simulink model "Distribution_v2"  (Simulink 7.9)
settings: Solver=VariableStepDiscrete  StartTime=0.0  StopTime=1000  RelTol=1e-3
libraries: simeventslib x35
(part 5 of 6)

== system Distribution_v2/Customer_15/Commodity_109 ==
  Clock : Clock
  Source : TimeBasedEntityGenerator  Distribution=Exponential  InitialSeed=18340  Mean=Mean  GenerateEntityAtSimulationStart=off
  Timed to Event Signal : TimedToEventSignal
  setAttribute : SetAttribute  AttributeName=Route|Origin|Destination|Start  AttributeFrom=Dialog|Dialog|Dialog|Signal port  AttributeValue="[15  20  11   0]|15|11|1"  AttributeTreatAsVector=0|1|1|1  EvaluatedAttributeValue="{[15  20  11   0];15;11;[]}"
      settings: InputPortMap=u3
  OUT_Commodity : PMIOPort  Port=1  Side=Right
  wires:
  Timed to Event Signal/1 -> setAttribute/1
  Clock/1 -> Timed to Event Signal/1
  connections:
  OUT_Commodity/RConn1 -- setAttribute/RConn1
  Source/RConn1 -- setAttribute/LConn1

== system Distribution_v2/Customer_15/Commodity_110 ==
  Clock : Clock
  Source : TimeBasedEntityGenerator  Distribution=Exponential  InitialSeed=18340  Mean=Mean  GenerateEntityAtSimulationStart=off
  Timed to Event Signal : TimedToEventSignal
  setAttribute : SetAttribute  AttributeName=Route|Origin|Destination|Start  AttributeFrom=Dialog|Dialog|Dialog|Signal port  AttributeValue="[15  20  22  12]|15|12|1"  AttributeTreatAsVector=0|1|1|1  EvaluatedAttributeValue="{[15  20  22  12];15;12;[]}"
      settings: InputPortMap=u3
  OUT_Commodity : PMIOPort  Port=1  Side=Right
  wires:
  Timed to Event Signal/1 -> setAttribute/1
  Clock/1 -> Timed to Event Signal/1
  connections:
  OUT_Commodity/RConn1 -- setAttribute/RConn1
  Source/RConn1 -- setAttribute/LConn1

== system Distribution_v2/Customer_15/Commodity_111 ==
  Clock : Clock
  Source : TimeBasedEntityGenerator  Distribution=Exponential  InitialSeed=18340  Mean=Mean  GenerateEntityAtSimulationStart=off
  Timed to Event Signal : TimedToEventSignal
  setAttribute : SetAttribute  AttributeName=Route|Origin|Destination|Start  AttributeFrom=Dialog|Dialog|Dialog|Signal port  AttributeValue="[15  20  22  13]|15|13|1"  AttributeTreatAsVector=0|1|1|1  EvaluatedAttributeValue="{[15  20  22  13];15;13;[]}"
      settings: InputPortMap=u3
  OUT_Commodity : PMIOPort  Port=1  Side=Right
  wires:
  Timed to Event Signal/1 -> setAttribute/1
  Clock/1 -> Timed to Event Signal/1
  connections:
  OUT_Commodity/RConn1 -- setAttribute/RConn1
  Source/RConn1 -- setAttribute/LConn1

== system Distribution_v2/Customer_2/Commodity_10 ==
  Clock : Clock
  Source : TimeBasedEntityGenerator  Distribution=Exponential  InitialSeed=18340  Mean=Mean  GenerateEntityAtSimulationStart=off
  Timed to Event Signal : TimedToEventSignal
  setAttribute : SetAttribute  AttributeName=Route|Origin|Destination|Start  AttributeFrom=Dialog|Dialog|Dialog|Signal port  AttributeValue="[2  18  22   1]|2|1|1"  AttributeTreatAsVector=0|1|1|1  EvaluatedAttributeValue="{[2  18  22   1];2;1;[]}"
      settings: InputPortMap=u3
  OUT_Commodity : PMIOPort  Port=1  Side=Right
  wires:
  Timed to Event Signal/1 -> setAttribute/1
  Clock/1 -> Timed to Event Signal/1
  connections:
  OUT_Commodity/RConn1 -- setAttribute/RConn1
  Source/RConn1 -- setAttribute/LConn1

== system Distribution_v2/Customer_2/Commodity_11 ==
  Clock : Clock
  Source : TimeBasedEntityGenerator  Distribution=Exponential  InitialSeed=18340  Mean=Mean  GenerateEntityAtSimulationStart=off
  Timed to Event Signal : TimedToEventSignal
  setAttribute : SetAttribute  AttributeName=Route|Origin|Destination|Start  AttributeFrom=Dialog|Dialog|Dialog|Signal port  AttributeValue="[2  18  20   3]|2|3|1"  AttributeTreatAsVector=0|1|1|1  EvaluatedAttributeValue="{[2  18  20   3];2;3;[]}"
      settings: InputPortMap=u3
  OUT_Commodity : PMIOPort  Port=1  Side=Right
  wires:
  Timed to Event Signal/1 -> setAttribute/1
  Clock/1 -> Timed to Event Signal/1
  connections:
  OUT_Commodity/RConn1 -- setAttribute/RConn1
  Source/RConn1 -- setAttribute/LConn1

== system Distribution_v2/Customer_2/Commodity_12 ==
  Clock : Clock
  Source : TimeBasedEntityGenerator  Distribution=Exponential  InitialSeed=18340  Mean=Mean  GenerateEntityAtSimulationStart=off
  Timed to Event Signal : TimedToEventSignal
  setAttribute : SetAttribute  AttributeName=Route|Origin|Destination|Start  AttributeFrom=Dialog|Dialog|Dialog|Signal port  AttributeValue="[2  18   4   0]|2|4|1"  AttributeTreatAsVector=0|1|1|1  EvaluatedAttributeValue="{[2  18   4   0];2;4;[]}"
      settings: InputPortMap=u3
  OUT_Commodity : PMIOPort  Port=1  Side=Right
  wires:
  Timed to Event Signal/1 -> setAttribute/1
  Clock/1 -> Timed to Event Signal/1
  connections:
  OUT_Commodity/RConn1 -- setAttribute/RConn1
  Source/RConn1 -- setAttribute/LConn1

== system Distribution_v2/Customer_2/Commodity_13 ==
  Clock : Clock
  Source : TimeBasedEntityGenerator  Distribution=Exponential  InitialSeed=18340  Mean=Mean  GenerateEntityAtSimulationStart=off
  Timed to Event Signal : TimedToEventSignal
  setAttribute : SetAttribute  AttributeName=Route|Origin|Destination|Start  AttributeFrom=Dialog|Dialog|Dialog|Signal port  AttributeValue="[2  18  22   5]|2|5|1"  AttributeTreatAsVector=0|1|1|1  EvaluatedAttributeValue="{[2  18  22   5];2;5;[]}"
      settings: InputPortMap=u3
  OUT_Commodity : PMIOPort  Port=1  Side=Right
  wires:
  Timed to Event Signal/1 -> setAttribute/1
  Clock/1 -> Timed to Event Signal/1
  connections:
  OUT_Commodity/RConn1 -- setAttribute/RConn1
  Source/RConn1 -- setAttribute/LConn1

== system Distribution_v2/Customer_2/Commodity_14 ==
  Clock : Clock
  Source : TimeBasedEntityGenerator  Distribution=Exponential  InitialSeed=18340  Mean=Mean  GenerateEntityAtSimulationStart=off
  Timed to Event Signal : TimedToEventSignal
  setAttribute : SetAttribute  AttributeName=Route|Origin|Destination|Start  AttributeFrom=Dialog|Dialog|Dialog|Signal port  AttributeValue="[2  18  22  10]|2|10|1"  AttributeTreatAsVector=0|1|1|1  EvaluatedAttributeValue="{[2  18  22  10];2;10;[]}"
      settings: InputPortMap=u3
  OUT_Commodity : PMIOPort  Port=1  Side=Right
  wires:
  Timed to Event Signal/1 -> setAttribute/1
  Clock/1 -> Timed to Event Signal/1
  connections:
  OUT_Commodity/RConn1 -- setAttribute/RConn1
  Source/RConn1 -- setAttribute/LConn1

== system Distribution_v2/Customer_2/Commodity_15 ==
  Clock : Clock
  Source : TimeBasedEntityGenerator  Distribution=Exponential  InitialSeed=18340  Mean=Mean  GenerateEntityAtSimulationStart=off
  Timed to Event Signal : TimedToEventSignal
  setAttribute : SetAttribute  AttributeName=Route|Origin|Destination|Start  AttributeFrom=Dialog|Dialog|Dialog|Signal port  AttributeValue="[2  18  22  12]|2|12|1"  AttributeTreatAsVector=0|1|1|1  EvaluatedAttributeValue="{[2  18  22  12];2;12;[]}"
      settings: InputPortMap=u3
  OUT_Commodity : PMIOPort  Port=1  Side=Right
  wires:
  Timed to Event Signal/1 -> setAttribute/1
  Clock/1 -> Timed to Event Signal/1
  connections:
  OUT_Commodity/RConn1 -- setAttribute/RConn1
  Source/RConn1 -- setAttribute/LConn1

== system Distribution_v2/Customer_2/Commodity_16 ==
  Clock : Clock
  Source : TimeBasedEntityGenerator  Distribution=Exponential  InitialSeed=18340  Mean=Mean  GenerateEntityAtSimulationStart=off
  Timed to Event Signal : TimedToEventSignal
  setAttribute : SetAttribute  AttributeName=Route|Origin|Destination|Start  AttributeFrom=Dialog|Dialog|Dialog|Signal port  AttributeValue="[2  18  22  13]|2|13|1"  AttributeTreatAsVector=0|1|1|1  EvaluatedAttributeValue="{[2  18  22  13];2;13;[]}"
      settings: InputPortMap=u3
  OUT_Commodity : PMIOPort  Port=1  Side=Right
  wires:
  Timed to Event Signal/1 -> setAttribute/1
  Clock/1 -> Timed to Event Signal/1
  connections:
  OUT_Commodity/RConn1 -- setAttribute/RConn1
  Source/RConn1 -- setAttribute/LConn1

== system Distribution_v2/Customer_3/Commodity_17 ==
  Clock : Clock
  Source : TimeBasedEntityGenerator  Distribution=Exponential  InitialSeed=18340  Mean=Mean  GenerateEntityAtSimulationStart=off
  Timed to Event Signal : TimedToEventSignal
  setAttribute : SetAttribute  AttributeName=Route|Origin|Destination|Start  AttributeFrom=Dialog|Dialog|Dialog|Signal port  AttributeValue="[3  20  18   2]|3|2|1"  AttributeTreatAsVector=0|1|1|1  EvaluatedAttributeValue="{[3  20  18   2];3;2;[]}"
      settings: InputPortMap=u3
  OUT_Commodity : PMIOPort  Port=1  Side=Right
  wires:
  Timed to Event Signal/1 -> setAttribute/1
  Clock/1 -> Timed to Event Signal/1
  connections:
  OUT_Commodity/RConn1 -- setAttribute/RConn1
  Source/RConn1 -- setAttribute/LConn1

== system Distribution_v2/Customer_3/Commodity_18 ==
  Clock : Clock
  Source : TimeBasedEntityGenerator  Distribution=Exponential  InitialSeed=18340  Mean=Mean  GenerateEntityAtSimulationStart=off
  Timed to Event Signal : TimedToEventSignal
  setAttribute : SetAttribute  AttributeName=Route|Origin|Destination|Start  AttributeFrom=Dialog|Dialog|Dialog|Signal port  AttributeValue="[3  20  18   4]|3|4|1"  AttributeTreatAsVector=0|1|1|1  EvaluatedAttributeValue="{[3  20  18   4];3;4;[]}"
      settings: InputPortMap=u3
  OUT_Commodity : PMIOPort  Port=1  Side=Right
  wires:
  Timed to Event Signal/1 -> setAttribute/1
  Clock/1 -> Timed to Event Signal/1
  connections:
  OUT_Commodity/RConn1 -- setAttribute/RConn1
  Source/RConn1 -- setAttribute/LConn1

== system Distribution_v2/Customer_3/Commodity_19 ==
  Clock : Clock
  Source : TimeBasedEntityGenerator  Distribution=Exponential  InitialSeed=18340  Mean=Mean  GenerateEntityAtSimulationStart=off
  Timed to Event Signal : TimedToEventSignal
  setAttribute : SetAttribute  AttributeName=Route|Origin|Destination|Start  AttributeFrom=Dialog|Dialog|Dialog|Signal port  AttributeValue="[3  20  22   5]|3|5|1"  AttributeTreatAsVector=0|1|1|1  EvaluatedAttributeValue="{[3  20  22   5];3;5;[]}"
      settings: InputPortMap=u3
  OUT_Commodity : PMIOPort  Port=1  Side=Right
  wires:
  Timed to Event Signal/1 -> setAttribute/1
  Clock/1 -> Timed to Event Signal/1
  connections:
  OUT_Commodity/RConn1 -- setAttribute/RConn1
  Source/RConn1 -- setAttribute/LConn1

== system Distribution_v2/Customer_3/Commodity_20 ==
  Clock : Clock
  Source : TimeBasedEntityGenerator  Distribution=Exponential  InitialSeed=18340  Mean=Mean  GenerateEntityAtSimulationStart=off
  Timed to Event Signal : TimedToEventSignal
  setAttribute : SetAttribute  AttributeName=Route|Origin|Destination|Start  AttributeFrom=Dialog|Dialog|Dialog|Signal port  AttributeValue="[3  20   7   0]|3|7|1"  AttributeTreatAsVector=0|1|1|1  EvaluatedAttributeValue="{[3  20   7   0];3;7;[]}"
      settings: InputPortMap=u3
  OUT_Commodity : PMIOPort  Port=1  Side=Right
  wires:
  Timed to Event Signal/1 -> setAttribute/1
  Clock/1 -> Timed to Event Signal/1
  connections:
  OUT_Commodity/RConn1 -- setAttribute/RConn1
  Source/RConn1 -- setAttribute/LConn1

== system Distribution_v2/Customer_3/Commodity_21 ==
  Clock : Clock
  Source : TimeBasedEntityGenerator  Distribution=Exponential  InitialSeed=18340  Mean=Mean  GenerateEntityAtSimulationStart=off
  Timed to Event Signal : TimedToEventSignal
  setAttribute : SetAttribute  AttributeName=Route|Origin|Destination|Start  AttributeFrom=Dialog|Dialog|Dialog|Signal port  AttributeValue="[3  20   8   0]|3|8|1"  AttributeTreatAsVector=0|1|1|1  EvaluatedAttributeValue="{[3  20   8   0];3;8;[]}"
      settings: InputPortMap=u3
  OUT_Commodity : PMIOPort  Port=1  Side=Right
  wires:
  Timed to Event Signal/1 -> setAttribute/1
  Clock/1 -> Timed to Event Signal/1
  connections:
  OUT_Commodity/RConn1 -- setAttribute/RConn1
  Source/RConn1 -- setAttribute/LConn1

== system Distribution_v2/Customer_3/Commodity_22 ==
  Clock : Clock
  Source : TimeBasedEntityGenerator  Distribution=Exponential  InitialSeed=18340  Mean=Mean  GenerateEntityAtSimulationStart=off
  Timed to Event Signal : TimedToEventSignal
  setAttribute : SetAttribute  AttributeName=Route|Origin|Destination|Start  AttributeFrom=Dialog|Dialog|Dialog|Signal port  AttributeValue="[3  20  18   9]|3|9|1"  AttributeTreatAsVector=0|1|1|1  EvaluatedAttributeValue="{[3  20  18   9];3;9;[]}"
      settings: InputPortMap=u3
  OUT_Commodity : PMIOPort  Port=1  Side=Right
  wires:
  Timed to Event Signal/1 -> setAttribute/1
  Clock/1 -> Timed to Event Signal/1
  connections:
  OUT_Commodity/RConn1 -- setAttribute/RConn1
  Source/RConn1 -- setAttribute/LConn1

== system Distribution_v2/Customer_3/Commodity_23 ==
  Clock : Clock
  Source : TimeBasedEntityGenerator  Distribution=Exponential  InitialSeed=18340  Mean=Mean  GenerateEntityAtSimulationStart=off
  Timed to Event Signal : TimedToEventSignal
  setAttribute : SetAttribute  AttributeName=Route|Origin|Destination|Start  AttributeFrom=Dialog|Dialog|Dialog|Signal port  AttributeValue="[3  20  22  12]|3|12|1"  AttributeTreatAsVector=0|1|1|1  EvaluatedAttributeValue="{[3  20  22  12];3;12;[]}"
      settings: InputPortMap=u3
  OUT_Commodity : PMIOPort  Port=1  Side=Right
  wires:
  Timed to Event Signal/1 -> setAttribute/1
  Clock/1 -> Timed to Event Signal/1
  connections:
  OUT_Commodity/RConn1 -- setAttribute/RConn1
  Source/RConn1 -- setAttribute/LConn1

== system Distribution_v2/Customer_3/Commodity_24 ==
  Clock : Clock
  Source : TimeBasedEntityGenerator  Distribution=Exponential  InitialSeed=18340  Mean=Mean  GenerateEntityAtSimulationStart=off
  Timed to Event Signal : TimedToEventSignal
  setAttribute : SetAttribute  AttributeName=Route|Origin|Destination|Start  AttributeFrom=Dialog|Dialog|Dialog|Signal port  AttributeValue="[3  20  22  13]|3|13|1"  AttributeTreatAsVector=0|1|1|1  EvaluatedAttributeValue="{[3  20  22  13];3;13;[]}"
      settings: InputPortMap=u3
  OUT_Commodity : PMIOPort  Port=1  Side=Right
  wires:
  Timed to Event Signal/1 -> setAttribute/1
  Clock/1 -> Timed to Event Signal/1
  connections:
  OUT_Commodity/RConn1 -- setAttribute/RConn1
  Source/RConn1 -- setAttribute/LConn1

== system Distribution_v2/Customer_3/Commodity_25 ==
  Clock : Clock
  Source : TimeBasedEntityGenerator  Distribution=Exponential  InitialSeed=18340  Mean=Mean  GenerateEntityAtSimulationStart=off
  Timed to Event Signal : TimedToEventSignal
  setAttribute : SetAttribute  AttributeName=Route|Origin|Destination|Start  AttributeFrom=Dialog|Dialog|Dialog|Signal port  AttributeValue="[3  20  14   0]|3|14|1"  AttributeTreatAsVector=0|1|1|1  EvaluatedAttributeValue="{[3  20  14   0];3;14;[]}"
      settings: InputPortMap=u3
  OUT_Commodity : PMIOPort  Port=1  Side=Right
  wires:
  Timed to Event Signal/1 -> setAttribute/1
  Clock/1 -> Timed to Event Signal/1
  connections:
  OUT_Commodity/RConn1 -- setAttribute/RConn1
  Source/RConn1 -- setAttribute/LConn1

== system Distribution_v2/Customer_4/Commodity_26 ==
  Clock : Clock
  Source : TimeBasedEntityGenerator  Distribution=Exponential  InitialSeed=18340  Mean=Mean  GenerateEntityAtSimulationStart=off
  Timed to Event Signal : TimedToEventSignal
  setAttribute : SetAttribute  AttributeName=Route|Origin|Destination|Start  AttributeFrom=Dialog|Dialog|Dialog|Signal port  AttributeValue="[4  18   2   0]|4|2|1"  AttributeTreatAsVector=0|1|1|1  EvaluatedAttributeValue="{[4  18   2   0];4;2;[]}"
      settings: InputPortMap=u3
  OUT_Commodity : PMIOPort  Port=1  Side=Right
  wires:
  Timed to Event Signal/1 -> setAttribute/1
  Clock/1 -> Timed to Event Signal/1
  connections:
  OUT_Commodity/RConn1 -- setAttribute/RConn1
  Source/RConn1 -- setAttribute/LConn1

== system Distribution_v2/Customer_4/Commodity_27 ==
  Clock : Clock
  Source : TimeBasedEntityGenerator  Distribution=Exponential  InitialSeed=18340  Mean=Mean  GenerateEntityAtSimulationStart=off
  Timed to Event Signal : TimedToEventSignal
  setAttribute : SetAttribute  AttributeName=Route|Origin|Destination|Start  AttributeFrom=Dialog|Dialog|Dialog|Signal port  AttributeValue="[4  18  20   3]|4|3|1"  AttributeTreatAsVector=0|1|1|1  EvaluatedAttributeValue="{[4  18  20   3];4;3;[]}"
      settings: InputPortMap=u3
  OUT_Commodity : PMIOPort  Port=1  Side=Right
  wires:
  Timed to Event Signal/1 -> setAttribute/1
  Clock/1 -> Timed to Event Signal/1
  connections:
  OUT_Commodity/RConn1 -- setAttribute/RConn1
  Source/RConn1 -- setAttribute/LConn1

== system Distribution_v2/Customer_4/Commodity_28 ==
  Clock : Clock
  Source : TimeBasedEntityGenerator  Distribution=Exponential  InitialSeed=18340  Mean=Mean  GenerateEntityAtSimulationStart=off
  Timed to Event Signal : TimedToEventSignal
  setAttribute : SetAttribute  AttributeName=Route|Origin|Destination|Start  AttributeFrom=Dialog|Dialog|Dialog|Signal port  AttributeValue="[4  18  22   5]|4|5|1"  AttributeTreatAsVector=0|1|1|1  EvaluatedAttributeValue="{[4  18  22   5];4;5;[]}"
      settings: InputPortMap=u3
  OUT_Commodity : PMIOPort  Port=1  Side=Right
  wires:
  Timed to Event Signal/1 -> setAttribute/1
  Clock/1 -> Timed to Event Signal/1
  connections:
  OUT_Commodity/RConn1 -- setAttribute/RConn1
  Source/RConn1 -- setAttribute/LConn1

== system Distribution_v2/Customer_4/Commodity_29 ==
  Clock : Clock
  Source : TimeBasedEntityGenerator  Distribution=Exponential  InitialSeed=18340  Mean=Mean  GenerateEntityAtSimulationStart=off
  Timed to Event Signal : TimedToEventSignal
  setAttribute : SetAttribute  AttributeName=Route|Origin|Destination|Start  AttributeFrom=Dialog|Dialog|Dialog|Signal port  AttributeValue="[4  18  20   8]|4|8|1"  AttributeTreatAsVector=0|1|1|1  EvaluatedAttributeValue="{[4  18  20   8];4;8;[]}"
      settings: InputPortMap=u3
  OUT_Commodity : PMIOPort  Port=1  Side=Right
  wires:
  Timed to Event Signal/1 -> setAttribute/1
  Clock/1 -> Timed to Event Signal/1
  connections:
  OUT_Commodity/RConn1 -- setAttribute/RConn1
  Source/RConn1 -- setAttribute/LConn1

== system Distribution_v2/Customer_4/Commodity_30 ==
  Clock : Clock
  Source : TimeBasedEntityGenerator  Distribution=Exponential  InitialSeed=18340  Mean=Mean  GenerateEntityAtSimulationStart=off
  Timed to Event Signal : TimedToEventSignal
  setAttribute : SetAttribute  AttributeName=Route|Origin|Destination|Start  AttributeFrom=Dialog|Dialog|Dialog|Signal port  AttributeValue="[4  18   9   0]|4|9|1"  AttributeTreatAsVector=0|1|1|1  EvaluatedAttributeValue="{[4  18   9   0];4;9;[]}"
      settings: InputPortMap=u3
  OUT_Commodity : PMIOPort  Port=1  Side=Right
  wires:
  Timed to Event Signal/1 -> setAttribute/1
  Clock/1 -> Timed to Event Signal/1
  connections:
  OUT_Commodity/RConn1 -- setAttribute/RConn1
  Source/RConn1 -- setAttribute/LConn1

== system Distribution_v2/Customer_4/Commodity_31 ==
  Clock : Clock
  Source : TimeBasedEntityGenerator  Distribution=Exponential  InitialSeed=18340  Mean=Mean  GenerateEntityAtSimulationStart=off
  Timed to Event Signal : TimedToEventSignal
  setAttribute : SetAttribute  AttributeName=Route|Origin|Destination|Start  AttributeFrom=Dialog|Dialog|Dialog|Signal port  AttributeValue="[4  18  22  10]|4|10|1"  AttributeTreatAsVector=0|1|1|1  EvaluatedAttributeValue="{[4  18  22  10];4;10;[]}"
      settings: InputPortMap=u3
  OUT_Commodity : PMIOPort  Port=1  Side=Right
  wires:
  Timed to Event Signal/1 -> setAttribute/1
  Clock/1 -> Timed to Event Signal/1
  connections:
  OUT_Commodity/RConn1 -- setAttribute/RConn1
  Source/RConn1 -- setAttribute/LConn1

== system Distribution_v2/Customer_4/Commodity_32 ==
  Clock : Clock
  Source : TimeBasedEntityGenerator  Distribution=Exponential  InitialSeed=18340  Mean=Mean  GenerateEntityAtSimulationStart=off
  Timed to Event Signal : TimedToEventSignal
  setAttribute : SetAttribute  AttributeName=Route|Origin|Destination|Start  AttributeFrom=Dialog|Dialog|Dialog|Signal port  AttributeValue="[4  18  20  11]|4|11|1"  AttributeTreatAsVector=0|1|1|1  EvaluatedAttributeValue="{[4  18  20  11];4;11;[]}"
      settings: InputPortMap=u3
  OUT_Commodity : PMIOPort  Port=1  Side=Right
  wires:
  Timed to Event Signal/1 -> setAttribute/1
  Clock/1 -> Timed to Event Signal/1
  connections:
  OUT_Commodity/RConn1 -- setAttribute/RConn1
  Source/RConn1 -- setAttribute/LConn1

== system Distribution_v2/Customer_4/Commodity_33 ==
  Clock : Clock
  Source : TimeBasedEntityGenerator  Distribution=Exponential  InitialSeed=18340  Mean=Mean  GenerateEntityAtSimulationStart=off
  Timed to Event Signal : TimedToEventSignal
  setAttribute : SetAttribute  AttributeName=Route|Origin|Destination|Start  AttributeFrom=Dialog|Dialog|Dialog|Signal port  AttributeValue="[4  18  22  12]|4|12|1"  AttributeTreatAsVector=0|1|1|1  EvaluatedAttributeValue="{[4  18  22  12];4;12;[]}"
      settings: InputPortMap=u3
  OUT_Commodity : PMIOPort  Port=1  Side=Right
  wires:
  Timed to Event Signal/1 -> setAttribute/1
  Clock/1 -> Timed to Event Signal/1
  connections:
  OUT_Commodity/RConn1 -- setAttribute/RConn1
  Source/RConn1 -- setAttribute/LConn1

== system Distribution_v2/Customer_5/Commodity_34 ==
  Clock : Clock
  Source : TimeBasedEntityGenerator  Distribution=Exponential  InitialSeed=18340  Mean=Mean  GenerateEntityAtSimulationStart=off
  Timed to Event Signal : TimedToEventSignal
  setAttribute : SetAttribute  AttributeName=Route|Origin|Destination|Start  AttributeFrom=Dialog|Dialog|Dialog|Signal port  AttributeValue="[5  22   1   0]|5|1|1"  AttributeTreatAsVector=0|1|1|1  EvaluatedAttributeValue="{[5  22   1   0];5;1;[]}"
      settings: InputPortMap=u3
  OUT_Commodity : PMIOPort  Port=1  Side=Right
  wires:
  Timed to Event Signal/1 -> setAttribute/1
  Clock/1 -> Timed to Event Signal/1
  connections:
  OUT_Commodity/RConn1 -- setAttribute/RConn1
  Source/RConn1 -- setAttribute/LConn1

== system Distribution_v2/Customer_5/Commodity_35 ==
  Clock : Clock
  Source : TimeBasedEntityGenerator  Distribution=Exponential  InitialSeed=18340  Mean=Mean  GenerateEntityAtSimulationStart=off
  Timed to Event Signal : TimedToEventSignal
  setAttribute : SetAttribute  AttributeName=Route|Origin|Destination|Start  AttributeFrom=Dialog|Dialog|Dialog|Signal port  AttributeValue="[5  22  20   3]|5|3|1"  AttributeTreatAsVector=0|1|1|1  EvaluatedAttributeValue="{[5  22  20   3];5;3;[]}"
      settings: InputPortMap=u3
  OUT_Commodity : PMIOPort  Port=1  Side=Right
  wires:
  Timed to Event Signal/1 -> setAttribute/1
  Clock/1 -> Timed to Event Signal/1
  connections:
  OUT_Commodity/RConn1 -- setAttribute/RConn1
  Source/RConn1 -- setAttribute/LConn1

== system Distribution_v2/Customer_5/Commodity_36 ==
  Clock : Clock
  Source : TimeBasedEntityGenerator  Distribution=Exponential  InitialSeed=18340  Mean=Mean  GenerateEntityAtSimulationStart=off
  Timed to Event Signal : TimedToEventSignal
  setAttribute : SetAttribute  AttributeName=Route|Origin|Destination|Start  AttributeFrom=Dialog|Dialog|Dialog|Signal port  AttributeValue="[5  22  18   4]|5|4|1"  AttributeTreatAsVector=0|1|1|1  EvaluatedAttributeValue="{[5  22  18   4];5;4;[]}"
      settings: InputPortMap=u3
  OUT_Commodity : PMIOPort  Port=1  Side=Right
  wires:
  Timed to Event Signal/1 -> setAttribute/1
  Clock/1 -> Timed to Event Signal/1
  connections:
  OUT_Commodity/RConn1 -- setAttribute/RConn1
  Source/RConn1 -- setAttribute/LConn1

== system Distribution_v2/Customer_5/Commodity_37 ==
  Clock : Clock
  Source : TimeBasedEntityGenerator  Distribution=Exponential  InitialSeed=18340  Mean=Mean  GenerateEntityAtSimulationStart=off
  Timed to Event Signal : TimedToEventSignal
  setAttribute : SetAttribute  AttributeName=Route|Origin|Destination|Start  AttributeFrom=Dialog|Dialog|Dialog|Signal port  AttributeValue="[5  22  18   6]|5|6|1"  AttributeTreatAsVector=0|1|1|1  EvaluatedAttributeValue="{[5  22  18   6];5;6;[]}"
      settings: InputPortMap=u3
  OUT_Commodity : PMIOPort  Port=1  Side=Right
  wires:
  Timed to Event Signal/1 -> setAttribute/1
  Clock/1 -> Timed to Event Signal/1
  connections:
  OUT_Commodity/RConn1 -- setAttribute/RConn1
  Source/RConn1 -- setAttribute/LConn1

== system Distribution_v2/Customer_5/Commodity_38 ==
  Clock : Clock
  Source : TimeBasedEntityGenerator  Distribution=Exponential  InitialSeed=18340  Mean=Mean  GenerateEntityAtSimulationStart=off
  Timed to Event Signal : TimedToEventSignal
  setAttribute : SetAttribute  AttributeName=Route|Origin|Destination|Start  AttributeFrom=Dialog|Dialog|Dialog|Signal port  AttributeValue="[5  22  20   7]|5|7|1"  AttributeTreatAsVector=0|1|1|1  EvaluatedAttributeValue="{[5  22  20   7];5;7;[]}"
      settings: InputPortMap=u3
  OUT_Commodity : PMIOPort  Port=1  Side=Right
  wires:
  Timed to Event Signal/1 -> setAttribute/1
  Clock/1 -> Timed to Event Signal/1
  connections:
  OUT_Commodity/RConn1 -- setAttribute/RConn1
  Source/RConn1 -- setAttribute/LConn1

== system Distribution_v2/Customer_5/Commodity_39 ==
  Clock : Clock
  Source : TimeBasedEntityGenerator  Distribution=Exponential  InitialSeed=18340  Mean=Mean  GenerateEntityAtSimulationStart=off
  Timed to Event Signal : TimedToEventSignal
  setAttribute : SetAttribute  AttributeName=Route|Origin|Destination|Start  AttributeFrom=Dialog|Dialog|Dialog|Signal port  AttributeValue="[5  22  20   8]|5|8|1"  AttributeTreatAsVector=0|1|1|1  EvaluatedAttributeValue="{[5  22  20   8];5;8;[]}"
      settings: InputPortMap=u3
  OUT_Commodity : PMIOPort  Port=1  Side=Right
  wires:
  Timed to Event Signal/1 -> setAttribute/1
  Clock/1 -> Timed to Event Signal/1
  connections:
  OUT_Commodity/RConn1 -- setAttribute/RConn1
  Source/RConn1 -- setAttribute/LConn1

== system Distribution_v2/Customer_5/Commodity_40 ==
  Clock : Clock
  Source : TimeBasedEntityGenerator  Distribution=Exponential  InitialSeed=18340  Mean=Mean  GenerateEntityAtSimulationStart=off
  Timed to Event Signal : TimedToEventSignal
  setAttribute : SetAttribute  AttributeName=Route|Origin|Destination|Start  AttributeFrom=Dialog|Dialog|Dialog|Signal port  AttributeValue="[5  22  20  11]|5|11|1"  AttributeTreatAsVector=0|1|1|1  EvaluatedAttributeValue="{[5  22  20  11];5;11;[]}"
      settings: InputPortMap=u3
  OUT_Commodity : PMIOPort  Port=1  Side=Right
  wires:
  Timed to Event Signal/1 -> setAttribute/1
  Clock/1 -> Timed to Event Signal/1
  connections:
  OUT_Commodity/RConn1 -- setAttribute/RConn1
  Source/RConn1 -- setAttribute/LConn1

== system Distribution_v2/Customer_5/Commodity_41 ==
  Clock : Clock
  Source : TimeBasedEntityGenerator  Distribution=Exponential  InitialSeed=18340  Mean=Mean  GenerateEntityAtSimulationStart=off
  Timed to Event Signal : TimedToEventSignal
  setAttribute : SetAttribute  AttributeName=Route|Origin|Destination|Start  AttributeFrom=Dialog|Dialog|Dialog|Signal port  AttributeValue="[5  22  12   0]|5|12|1"  AttributeTreatAsVector=0|1|1|1  EvaluatedAttributeValue="{[5  22  12   0];5;12;[]}"
      settings: InputPortMap=u3
  OUT_Commodity : PMIOPort  Port=1  Side=Right
  wires:
  Timed to Event Signal/1 -> setAttribute/1
  Clock/1 -> Timed to Event Signal/1
  connections:
  OUT_Commodity/RConn1 -- setAttribute/RConn1
  Source/RConn1 -- setAttribute/LConn1

== system Distribution_v2/Customer_5/Commodity_42 ==
  Clock : Clock
  Source : TimeBasedEntityGenerator  Distribution=Exponential  InitialSeed=18340  Mean=Mean  GenerateEntityAtSimulationStart=off
  Timed to Event Signal : TimedToEventSignal
  setAttribute : SetAttribute  AttributeName=Route|Origin|Destination|Start  AttributeFrom=Dialog|Dialog|Dialog|Signal port  AttributeValue="[5  22  13   0]|5|13|1"  AttributeTreatAsVector=0|1|1|1  EvaluatedAttributeValue="{[5  22  13   0];5;13;[]}"
      settings: InputPortMap=u3
  OUT_Commodity : PMIOPort  Port=1  Side=Right
  wires:
  Timed to Event Signal/1 -> setAttribute/1
  Clock/1 -> Timed to Event Signal/1
  connections:
  OUT_Commodity/RConn1 -- setAttribute/RConn1
  Source/RConn1 -- setAttribute/LConn1

== system Distribution_v2/Customer_5/Commodity_43 ==
  Clock : Clock
  Source : TimeBasedEntityGenerator  Distribution=Exponential  InitialSeed=18340  Mean=Mean  GenerateEntityAtSimulationStart=off
  Timed to Event Signal : TimedToEventSignal
  setAttribute : SetAttribute  AttributeName=Route|Origin|Destination|Start  AttributeFrom=Dialog|Dialog|Dialog|Signal port  AttributeValue="[5  22  20  15]|5|15|1"  AttributeTreatAsVector=0|1|1|1  EvaluatedAttributeValue="{[5  22  20  15];5;15;[]}"
      settings: InputPortMap=u3
  OUT_Commodity : PMIOPort  Port=1  Side=Right
  wires:
  Timed to Event Signal/1 -> setAttribute/1
  Clock/1 -> Timed to Event Signal/1
  connections:
  OUT_Commodity/RConn1 -- setAttribute/RConn1
  Source/RConn1 -- setAttribute/LConn1

== system Distribution_v2/Customer_6/Commodity_44 ==
  Clock : Clock
  Source : TimeBasedEntityGenerator  Distribution=Exponential  InitialSeed=18340  Mean=Mean  GenerateEntityAtSimulationStart=off
  Timed to Event Signal : TimedToEventSignal
  setAttribute : SetAttribute  AttributeName=Route|Origin|Destination|Start  AttributeFrom=Dialog|Dialog|Dialog|Signal port  AttributeValue="[6  18  22   1]|6|1|1"  AttributeTreatAsVector=0|1|1|1  EvaluatedAttributeValue="{[6  18  22   1];6;1;[]}"
      settings: InputPortMap=u3
  OUT_Commodity : PMIOPort  Port=1  Side=Right
  wires:
  Timed to Event Signal/1 -> setAttribute/1
  Clock/1 -> Timed to Event Signal/1
  connections:
  OUT_Commodity/RConn1 -- setAttribute/RConn1
  Source/RConn1 -- setAttribute/LConn1

== system Distribution_v2/Customer_6/Commodity_45 ==
  Clock : Clock
  Source : TimeBasedEntityGenerator  Distribution=Exponential  InitialSeed=18340  Mean=Mean  GenerateEntityAtSimulationStart=off
  Timed to Event Signal : TimedToEventSignal
  setAttribute : SetAttribute  AttributeName=Route|Origin|Destination|Start  AttributeFrom=Dialog|Dialog|Dialog|Signal port  AttributeValue="[6  18   2   0]|6|2|1"  AttributeTreatAsVector=0|1|1|1  EvaluatedAttributeValue="{[6  18   2   0];6;2;[]}"
      settings: InputPortMap=u3
  OUT_Commodity : PMIOPort  Port=1  Side=Right
  wires:
  Timed to Event Signal/1 -> setAttribute/1
  Clock/1 -> Timed to Event Signal/1
  connections:
  OUT_Commodity/RConn1 -- setAttribute/RConn1
  Source/RConn1 -- setAttribute/LConn1

== system Distribution_v2/Customer_6/Commodity_46 ==
  Clock : Clock
  Source : TimeBasedEntityGenerator  Distribution=Exponential  InitialSeed=18340  Mean=Mean  GenerateEntityAtSimulationStart=off
  Timed to Event Signal : TimedToEventSignal
  setAttribute : SetAttribute  AttributeName=Route|Origin|Destination|Start  AttributeFrom=Dialog|Dialog|Dialog|Signal port  AttributeValue="[6  18  22   5]|6|5|1"  AttributeTreatAsVector=0|1|1|1  EvaluatedAttributeValue="{[6  18  22   5];6;5;[]}"
      settings: InputPortMap=u3
  OUT_Commodity : PMIOPort  Port=1  Side=Right
  wires:
  Timed to Event Signal/1 -> setAttribute/1
  Clock/1 -> Timed to Event Signal/1
  connections:
  OUT_Commodity/RConn1 -- setAttribute/RConn1
  Source/RConn1 -- setAttribute/LConn1

== system Distribution_v2/Customer_6/Commodity_47 ==
  Clock : Clock
  Source : TimeBasedEntityGenerator  Distribution=Exponential  InitialSeed=18340  Mean=Mean  GenerateEntityAtSimulationStart=off
  Timed to Event Signal : TimedToEventSignal
  setAttribute : SetAttribute  AttributeName=Route|Origin|Destination|Start  AttributeFrom=Dialog|Dialog|Dialog|Signal port  AttributeValue="[6  18  20   7]|6|7|1"  AttributeTreatAsVector=0|1|1|1  EvaluatedAttributeValue="{[6  18  20   7];6;7;[]}"
      settings: InputPortMap=u3
  OUT_Commodity : PMIOPort  Port=1  Side=Right
  wires:
  Timed to Event Signal/1 -> setAttribute/1
  Clock/1 -> Timed to Event Signal/1
  connections:
  OUT_Commodity/RConn1 -- setAttribute/RConn1
  Source/RConn1 -- setAttribute/LConn1

== system Distribution_v2/Customer_6/Commodity_48 ==
  Clock : Clock
  Source : TimeBasedEntityGenerator  Distribution=Exponential  InitialSeed=18340  Mean=Mean  GenerateEntityAtSimulationStart=off
  Timed to Event Signal : TimedToEventSignal
  setAttribute : SetAttribute  AttributeName=Route|Origin|Destination|Start  AttributeFrom=Dialog|Dialog|Dialog|Signal port  AttributeValue="[6  18  20   8]|6|8|1"  AttributeTreatAsVector=0|1|1|1  EvaluatedAttributeValue="{[6  18  20   8];6;8;[]}"
      settings: InputPortMap=u3
  OUT_Commodity : PMIOPort  Port=1  Side=Right
  wires:
  Timed to Event Signal/1 -> setAttribute/1
  Clock/1 -> Timed to Event Signal/1
  connections:
  OUT_Commodity/RConn1 -- setAttribute/RConn1
  Source/RConn1 -- setAttribute/LConn1

== system Distribution_v2/Customer_6/Commodity_49 ==
  Clock : Clock
  Source : TimeBasedEntityGenerator  Distribution=Exponential  InitialSeed=18340  Mean=Mean  GenerateEntityAtSimulationStart=off
  Timed to Event Signal : TimedToEventSignal
  setAttribute : SetAttribute  AttributeName=Route|Origin|Destination|Start  AttributeFrom=Dialog|Dialog|Dialog|Signal port  AttributeValue="[6  18   9   0]|6|9|1"  AttributeTreatAsVector=0|1|1|1  EvaluatedAttributeValue="{[6  18   9   0];6;9;[]}"
      settings: InputPortMap=u3
  OUT_Commodity : PMIOPort  Port=1  Side=Right
  wires:
  Timed to Event Signal/1 -> setAttribute/1
  Clock/1 -> Timed to Event Signal/1
  connections:
  OUT_Commodity/RConn1 -- setAttribute/RConn1
  Source/RConn1 -- setAttribute/LConn1

== system Distribution_v2/Customer_6/Commodity_50 ==
  Clock : Clock
  Source : TimeBasedEntityGenerator  Distribution=Exponential  InitialSeed=18340  Mean=Mean  GenerateEntityAtSimulationStart=off
  Timed to Event Signal : TimedToEventSignal
  setAttribute : SetAttribute  AttributeName=Route|Origin|Destination|Start  AttributeFrom=Dialog|Dialog|Dialog|Signal port  AttributeValue="[6  18  22  12]|6|12|1"  AttributeTreatAsVector=0|1|1|1  EvaluatedAttributeValue="{[6  18  22  12];6;12;[]}"
      settings: InputPortMap=u3
  OUT_Commodity : PMIOPort  Port=1  Side=Right
  wires:
  Timed to Event Signal/1 -> setAttribute/1
  Clock/1 -> Timed to Event Signal/1
  connections:
  OUT_Commodity/RConn1 -- setAttribute/RConn1
  Source/RConn1 -- setAttribute/LConn1

== system Distribution_v2/Customer_6/Commodity_51 ==
  Clock : Clock
  Source : TimeBasedEntityGenerator  Distribution=Exponential  InitialSeed=18340  Mean=Mean  GenerateEntityAtSimulationStart=off
  Timed to Event Signal : TimedToEventSignal
  setAttribute : SetAttribute  AttributeName=Route|Origin|Destination|Start  AttributeFrom=Dialog|Dialog|Dialog|Signal port  AttributeValue="[6  18  22  13]|6|13|1"  AttributeTreatAsVector=0|1|1|1  EvaluatedAttributeValue="{[6  18  22  13];6;13;[]}"
      settings: InputPortMap=u3
  OUT_Commodity : PMIOPort  Port=1  Side=Right
  wires:
  Timed to Event Signal/1 -> setAttribute/1
  Clock/1 -> Timed to Event Signal/1
  connections:
  OUT_Commodity/RConn1 -- setAttribute/RConn1
  Source/RConn1 -- setAttribute/LConn1

== system Distribution_v2/Customer_6/Commodity_52 ==
  Clock : Clock
  Source : TimeBasedEntityGenerator  Distribution=Exponential  InitialSeed=18340  Mean=Mean  GenerateEntityAtSimulationStart=off
  Timed to Event Signal : TimedToEventSignal
  setAttribute : SetAttribute  AttributeName=Route|Origin|Destination|Start  AttributeFrom=Dialog|Dialog|Dialog|Signal port  AttributeValue="[6  18  20  14]|6|14|1"  AttributeTreatAsVector=0|1|1|1  EvaluatedAttributeValue="{[6  18  20  14];6;14;[]}"
      settings: InputPortMap=u3
  OUT_Commodity : PMIOPort  Port=1  Side=Right
  wires:
  Timed to Event Signal/1 -> setAttribute/1
  Clock/1 -> Timed to Event Signal/1
  connections:
  OUT_Commodity/RConn1 -- setAttribute/RConn1
  Source/RConn1 -- setAttribute/LConn1

== system Distribution_v2/Customer_6/Commodity_53 ==
  Clock : Clock
  Source : TimeBasedEntityGenerator  Distribution=Exponential  InitialSeed=18340  Mean=Mean  GenerateEntityAtSimulationStart=off
  Timed to Event Signal : TimedToEventSignal
  setAttribute : SetAttribute  AttributeName=Route|Origin|Destination|Start  AttributeFrom=Dialog|Dialog|Dialog|Signal port  AttributeValue="[6  18  20  15]|6|15|1"  AttributeTreatAsVector=0|1|1|1  EvaluatedAttributeValue="{[6  18  20  15];6;15;[]}"
      settings: InputPortMap=u3
  OUT_Commodity : PMIOPort  Port=1  Side=Right
  wires:
  Timed to Event Signal/1 -> setAttribute/1
  Clock/1 -> Timed to Event Signal/1
  connections:
  OUT_Commodity/RConn1 -- setAttribute/RConn1
  Source/RConn1 -- setAttribute/LConn1

== system Distribution_v2/Customer_7/Commodity_54 ==
  Clock : Clock
  Source : TimeBasedEntityGenerator  Distribution=Exponential  InitialSeed=18340  Mean=Mean  GenerateEntityAtSimulationStart=off
  Timed to Event Signal : TimedToEventSignal
  setAttribute : SetAttribute  AttributeName=Route|Origin|Destination|Start  AttributeFrom=Dialog|Dialog|Dialog|Signal port  AttributeValue="[7  20   3   0]|7|3|1"  AttributeTreatAsVector=0|1|1|1  EvaluatedAttributeValue="{[7  20   3   0];7;3;[]}"
      settings: InputPortMap=u3
  OUT_Commodity : PMIOPort  Port=1  Side=Right
  wires:
  Timed to Event Signal/1 -> setAttribute/1
  Clock/1 -> Timed to Event Signal/1
  connections:
  OUT_Commodity/RConn1 -- setAttribute/RConn1
  Source/RConn1 -- setAttribute/LConn1

== system Distribution_v2/Customer_7/Commodity_55 ==
  Clock : Clock
  Source : TimeBasedEntityGenerator  Distribution=Exponential  InitialSeed=18340  Mean=Mean  GenerateEntityAtSimulationStart=off
  Timed to Event Signal : TimedToEventSignal
  setAttribute : SetAttribute  AttributeName=Route|Origin|Destination|Start  AttributeFrom=Dialog|Dialog|Dialog|Signal port  AttributeValue="[7  20  22   5]|7|5|1"  AttributeTreatAsVector=0|1|1|1  EvaluatedAttributeValue="{[7  20  22   5];7;5;[]}"
      settings: InputPortMap=u3
  OUT_Commodity : PMIOPort  Port=1  Side=Right
  wires:
  Timed to Event Signal/1 -> setAttribute/1
  Clock/1 -> Timed to Event Signal/1
  connections:
  OUT_Commodity/RConn1 -- setAttribute/RConn1
  Source/RConn1 -- setAttribute/LConn1

== system Distribution_v2/Customer_7/Commodity_56 ==
  Clock : Clock
  Source : TimeBasedEntityGenerator  Distribution=Exponential  InitialSeed=18340  Mean=Mean  GenerateEntityAtSimulationStart=off
  Timed to Event Signal : TimedToEventSignal
  setAttribute : SetAttribute  AttributeName=Route|Origin|Destination|Start  AttributeFrom=Dialog|Dialog|Dialog|Signal port  AttributeValue="[7  20  18   6]|7|6|1"  AttributeTreatAsVector=0|1|1|1  EvaluatedAttributeValue="{[7  20  18   6];7;6;[]}"
      settings: InputPortMap=u3
  OUT_Commodity : PMIOPort  Port=1  Side=Right
  wires:
  Timed to Event Signal/1 -> setAttribute/1
  Clock/1 -> Timed to Event Signal/1
  connections:
  OUT_Commodity/RConn1 -- setAttribute/RConn1
  Source/RConn1 -- setAttribute/LConn1

== system Distribution_v2/Customer_7/Commodity_57 ==
  Clock : Clock
  Source : TimeBasedEntityGenerator  Distribution=Exponential  InitialSeed=18340  Mean=Mean  GenerateEntityAtSimulationStart=off
  Timed to Event Signal : TimedToEventSignal
  setAttribute : SetAttribute  AttributeName=Route|Origin|Destination|Start  AttributeFrom=Dialog|Dialog|Dialog|Signal port  AttributeValue="[7  20  22  13]|7|13|1"  AttributeTreatAsVector=0|1|1|1  EvaluatedAttributeValue="{[7  20  22  13];7;13;[]}"
      settings: InputPortMap=u3
  OUT_Commodity : PMIOPort  Port=1  Side=Right
  wires:
  Timed to Event Signal/1 -> setAttribute/1
  Clock/1 -> Timed to Event Signal/1
  connections:
  OUT_Commodity/RConn1 -- setAttribute/RConn1
  Source/RConn1 -- setAttribute/LConn1

== system Distribution_v2/Customer_7/Commodity_58 ==
  Clock : Clock
  Source : TimeBasedEntityGenerator  Distribution=Exponential  InitialSeed=18340  Mean=Mean  GenerateEntityAtSimulationStart=off
  Timed to Event Signal : TimedToEventSignal
  setAttribute : SetAttribute  AttributeName=Route|Origin|Destination|Start  AttributeFrom=Dialog|Dialog|Dialog|Signal port  AttributeValue="[7  20  15   0]|7|15|1"  AttributeTreatAsVector=0|1|1|1  EvaluatedAttributeValue="{[7  20  15   0];7;15;[]}"
      settings: InputPortMap=u3
  OUT_Commodity : PMIOPort  Port=1  Side=Right
  wires:
  Timed to Event Signal/1 -> setAttribute/1
  Clock/1 -> Timed to Event Signal/1
  connections:
  OUT_Commodity/RConn1 -- setAttribute/RConn1
  Source/RConn1 -- setAttribute/LConn1

== system Distribution_v2/Customer_8/Commodity_59 ==
  Clock : Clock
  Source : TimeBasedEntityGenerator  Distribution=Exponential  InitialSeed=18340  Mean=Mean  GenerateEntityAtSimulationStart=off
  Timed to Event Signal : TimedToEventSignal
  setAttribute : SetAttribute  AttributeName=Route|Origin|Destination|Start  AttributeFrom=Dialog|Dialog|Dialog|Signal port  AttributeValue="[8  20  22   5]|8|5|1"  AttributeTreatAsVector=0|1|1|1  EvaluatedAttributeValue="{[8  20  22   5];8;5;[]}"
      settings: InputPortMap=u3
  OUT_Commodity : PMIOPort  Port=1  Side=Right
  wires:
  Timed to Event Signal/1 -> setAttribute/1
  Clock/1 -> Timed to Event Signal/1
  connections:
  OUT_Commodity/RConn1 -- setAttribute/RConn1
  Source/RConn1 -- setAttribute/LConn1

== system Distribution_v2/Customer_8/Commodity_60 ==
  Clock : Clock
  Source : TimeBasedEntityGenerator  Distribution=Exponential  InitialSeed=18340  Mean=Mean  GenerateEntityAtSimulationStart=off
  Timed to Event Signal : TimedToEventSignal
  setAttribute : SetAttribute  AttributeName=Route|Origin|Destination|Start  AttributeFrom=Dialog|Dialog|Dialog|Signal port  AttributeValue="[8  20  18   6]|8|6|1"  AttributeTreatAsVector=0|1|1|1  EvaluatedAttributeValue="{[8  20  18   6];8;6;[]}"
      settings: InputPortMap=u3
  OUT_Commodity : PMIOPort  Port=1  Side=Right
  wires:
  Timed to Event Signal/1 -> setAttribute/1
  Clock/1 -> Timed to Event Signal/1
  connections:
  OUT_Commodity/RConn1 -- setAttribute/RConn1
  Source/RConn1 -- setAttribute/LConn1

== system Distribution_v2/Customer_8/Commodity_61 ==
  Clock : Clock
  Source : TimeBasedEntityGenerator  Distribution=Exponential  InitialSeed=18340  Mean=Mean  GenerateEntityAtSimulationStart=off
  Timed to Event Signal : TimedToEventSignal
  setAttribute : SetAttribute  AttributeName=Route|Origin|Destination|Start  AttributeFrom=Dialog|Dialog|Dialog|Signal port  AttributeValue="[8  20  18   9]|8|9|1"  AttributeTreatAsVector=0|1|1|1  EvaluatedAttributeValue="{[8  20  18   9];8;9;[]}"
      settings: InputPortMap=u3
  OUT_Commodity : PMIOPort  Port=1  Side=Right
  wires:
  Timed to Event Signal/1 -> setAttribute/1
  Clock/1 -> Timed to Event Signal/1
  connections:
  OUT_Commodity/RConn1 -- setAttribute/RConn1
  Source/RConn1 -- setAttribute/LConn1

== system Distribution_v2/Customer_8/Commodity_62 ==
  Clock : Clock
  Source : TimeBasedEntityGenerator  Distribution=Exponential  InitialSeed=18340  Mean=Mean  GenerateEntityAtSimulationStart=off
  Timed to Event Signal : TimedToEventSignal
  setAttribute : SetAttribute  AttributeName=Route|Origin|Destination|Start  AttributeFrom=Dialog|Dialog|Dialog|Signal port  AttributeValue="[8  20  22  10]|8|10|1"  AttributeTreatAsVector=0|1|1|1  EvaluatedAttributeValue="{[8  20  22  10];8;10;[]}"
      settings: InputPortMap=u3
  OUT_Commodity : PMIOPort  Port=1  Side=Right
  wires:
  Timed to Event Signal/1 -> setAttribute/1
  Clock/1 -> Timed to Event Signal/1
  connections:
  OUT_Commodity/RConn1 -- setAttribute/RConn1
  Source/RConn1 -- setAttribute/LConn1

== system Distribution_v2/Customer_8/Commodity_63 ==
  Clock : Clock
  Source : TimeBasedEntityGenerator  Distribution=Exponential  InitialSeed=18340  Mean=Mean  GenerateEntityAtSimulationStart=off
  Timed to Event Signal : TimedToEventSignal
  setAttribute : SetAttribute  AttributeName=Route|Origin|Destination|Start  AttributeFrom=Dialog|Dialog|Dialog|Signal port  AttributeValue="[8  20  11   0]|8|11|1"  AttributeTreatAsVector=0|1|1|1  EvaluatedAttributeValue="{[8  20  11   0];8;11;[]}"
      settings: InputPortMap=u3
  OUT_Commodity : PMIOPort  Port=1  Side=Right
  wires:
  Timed to Event Signal/1 -> setAttribute/1
  Clock/1 -> Timed to Event Signal/1
  connections:
  OUT_Commodity/RConn1 -- setAttribute/RConn1
  Source/RConn1 -- setAttribute/LConn1

== system Distribution_v2/Customer_8/Commodity_64 ==
  Clock : Clock
  Source : TimeBasedEntityGenerator  Distribution=Exponential  InitialSeed=18340  Mean=Mean  GenerateEntityAtSimulationStart=off
  Timed to Event Signal : TimedToEventSignal
  setAttribute : SetAttribute  AttributeName=Route|Origin|Destination|Start  AttributeFrom=Dialog|Dialog|Dialog|Signal port  AttributeValue="[8  20  22  13]|8|13|1"  AttributeTreatAsVector=0|1|1|1  EvaluatedAttributeValue="{[8  20  22  13];8;13;[]}"
      settings: InputPortMap=u3
  OUT_Commodity : PMIOPort  Port=1  Side=Right
  wires:
  Timed to Event Signal/1 -> setAttribute/1
  Clock/1 -> Timed to Event Signal/1
  connections:
  OUT_Commodity/RConn1 -- setAttribute/RConn1
  Source/RConn1 -- setAttribute/LConn1

== system Distribution_v2/Customer_9/Commodity_65 ==
  Clock : Clock
  Source : TimeBasedEntityGenerator  Distribution=Exponential  InitialSeed=18340  Mean=Mean  GenerateEntityAtSimulationStart=off
  Timed to Event Signal : TimedToEventSignal
  setAttribute : SetAttribute  AttributeName=Route|Origin|Destination|Start  AttributeFrom=Dialog|Dialog|Dialog|Signal port  AttributeValue="[9  18  22   1]|9|1|1"  AttributeTreatAsVector=0|1|1|1  EvaluatedAttributeValue="{[9  18  22   1];9;1;[]}"
      settings: InputPortMap=u3
  OUT_Commodity : PMIOPort  Port=1  Side=Right
  wires:
  Timed to Event Signal/1 -> setAttribute/1
  Clock/1 -> Timed to Event Signal/1
  connections:
  OUT_Commodity/RConn1 -- setAttribute/RConn1
  Source/RConn1 -- setAttribute/LConn1

== system Distribution_v2/Customer_9/Commodity_66 ==
  Clock : Clock
  Source : TimeBasedEntityGenerator  Distribution=Exponential  InitialSeed=18340  Mean=Mean  GenerateEntityAtSimulationStart=off
  Timed to Event Signal : TimedToEventSignal
  setAttribute : SetAttribute  AttributeName=Route|Origin|Destination|Start  AttributeFrom=Dialog|Dialog|Dialog|Signal port  AttributeValue="[9  18   2   0]|9|2|1"  AttributeTreatAsVector=0|1|1|1  EvaluatedAttributeValue="{[9  18   2   0];9;2;[]}"
      settings: InputPortMap=u3
  OUT_Commodity : PMIOPort  Port=1  Side=Right
  wires:
  Timed to Event Signal/1 -> setAttribute/1
  Clock/1 -> Timed to Event Signal/1
  connections:
  OUT_Commodity/RConn1 -- setAttribute/RConn1
  Source/RConn1 -- setAttribute/LConn1

== system Distribution_v2/Customer_9/Commodity_67 ==
  Clock : Clock
  Source : TimeBasedEntityGenerator  Distribution=Exponential  InitialSeed=18340  Mean=Mean  GenerateEntityAtSimulationStart=off
  Timed to Event Signal : TimedToEventSignal
  setAttribute : SetAttribute  AttributeName=Route|Origin|Destination|Start  AttributeFrom=Dialog|Dialog|Dialog|Signal port  AttributeValue="[9  18   4   0]|9|4|1"  AttributeTreatAsVector=0|1|1|1  EvaluatedAttributeValue="{[9  18   4   0];9;4;[]}"
      settings: InputPortMap=u3
  OUT_Commodity : PMIOPort  Port=1  Side=Right
  wires:
  Timed to Event Signal/1 -> setAttribute/1
  Clock/1 -> Timed to Event Signal/1
  connections:
  OUT_Commodity/RConn1 -- setAttribute/RConn1
  Source/RConn1 -- setAttribute/LConn1

== system Distribution_v2/Customer_9/Commodity_68 ==
  Clock : Clock
  Source : TimeBasedEntityGenerator  Distribution=Exponential  InitialSeed=18340  Mean=Mean  GenerateEntityAtSimulationStart=off
  Timed to Event Signal : TimedToEventSignal
  setAttribute : SetAttribute  AttributeName=Route|Origin|Destination|Start  AttributeFrom=Dialog|Dialog|Dialog|Signal port  AttributeValue="[9  18   6   0]|9|6|1"  AttributeTreatAsVector=0|1|1|1  EvaluatedAttributeValue="{[9  18   6   0];9;6;[]}"
      settings: InputPortMap=u3
  OUT_Commodity : PMIOPort  Port=1  Side=Right
  wires:
  Timed to Event Signal/1 -> setAttribute/1
  Clock/1 -> Timed to Event Signal/1
  connections:
  OUT_Commodity/RConn1 -- setAttribute/RConn1
  Source/RConn1 -- setAttribute/LConn1

== system Distribution_v2/Customer_9/Commodity_69 ==
  Clock : Clock
  Source : TimeBasedEntityGenerator  Distribution=Exponential  InitialSeed=18340  Mean=Mean  GenerateEntityAtSimulationStart=off
  Timed to Event Signal : TimedToEventSignal
  setAttribute : SetAttribute  AttributeName=Route|Origin|Destination|Start  AttributeFrom=Dialog|Dialog|Dialog|Signal port  AttributeValue="[9  18  20   7]|9|7|1"  AttributeTreatAsVector=0|1|1|1  EvaluatedAttributeValue="{[9  18  20   7];9;7;[]}"
      settings: InputPortMap=u3
  OUT_Commodity : PMIOPort  Port=1  Side=Right
  wires:
  Timed to Event Signal/1 -> setAttribute/1
  Clock/1 -> Timed to Event Signal/1
  connections:
  OUT_Commodity/RConn1 -- setAttribute/RConn1
  Source/RConn1 -- setAttribute/LConn1

== system Distribution_v2/Customer_9/Commodity_70 ==
  Clock : Clock
  Source : TimeBasedEntityGenerator  Distribution=Exponential  InitialSeed=18340  Mean=Mean  GenerateEntityAtSimulationStart=off
  Timed to Event Signal : TimedToEventSignal
  setAttribute : SetAttribute  AttributeName=Route|Origin|Destination|Start  AttributeFrom=Dialog|Dialog|Dialog|Signal port  AttributeValue="[9  18  20   8]|9|8|1"  AttributeTreatAsVector=0|1|1|1  EvaluatedAttributeValue="{[9  18  20   8];9;8;[]}"
      settings: InputPortMap=u3
  OUT_Commodity : PMIOPort  Port=1  Side=Right
  wires:
  Timed to Event Signal/1 -> setAttribute/1
  Clock/1 -> Timed to Event Signal/1
  connections:
  OUT_Commodity/RConn1 -- setAttribute/RConn1
  Source/RConn1 -- setAttribute/LConn1

== system Distribution_v2/Customer_9/Commodity_71 ==
  Clock : Clock
  Source : TimeBasedEntityGenerator  Distribution=Exponential  InitialSeed=18340  Mean=Mean  GenerateEntityAtSimulationStart=off
  Timed to Event Signal : TimedToEventSignal
  setAttribute : SetAttribute  AttributeName=Route|Origin|Destination|Start  AttributeFrom=Dialog|Dialog|Dialog|Signal port  AttributeValue="[9  18  22  10]|9|10|1"  AttributeTreatAsVector=0|1|1|1  EvaluatedAttributeValue="{[9  18  22  10];9;10;[]}"
      settings: InputPortMap=u3
  OUT_Commodity : PMIOPort  Port=1  Side=Right
  wires:
  Timed to Event Signal/1 -> setAttribute/1
  Clock/1 -> Timed to Event Signal/1
  connections:
  OUT_Commodity/RConn1 -- setAttribute/RConn1
  Source/RConn1 -- setAttribute/LConn1
